simulink model "ECU_AEMACE"  (R2021b)
settings: Solver=FixedStepDiscrete  StartTime=0.0  StopTime=inf  RelTol=1e-3
undefined symbols (not defined in the file or in its folder): IO682
libraries: speedgoatlib_IO682 x38, simulink x1
settings Model: Creator=ACH  LastModifiedBy=angel
settings SolverCC: ConcurrentTasks=on  PositivePriorityOrder=on
settings OptimizationCC: BlockReduction=off  OptimizeBlockIOStorage=off
settings DebuggingCC: TasksWithSamePriorityMsg=none
settings HardwareCC: ProdBitPerLong=64  ProdLongLongMode=on  ProdHWDeviceType=Intel->x86-64 (Linux 64)
settings RTWCC: Description=Simulink Real-Time  SystemTargetFile=slrealtime.tlc  TemplateMakefile=slrealtime_default_tmf  Toolchain=Simulink Real-Time Toolchain  BuildConfiguration=Faster Runs  CodeExecutionProfiling=on  TargetLang=C++
settings SimulinkRealTimeTargetCC: UseGCCFastMath=on

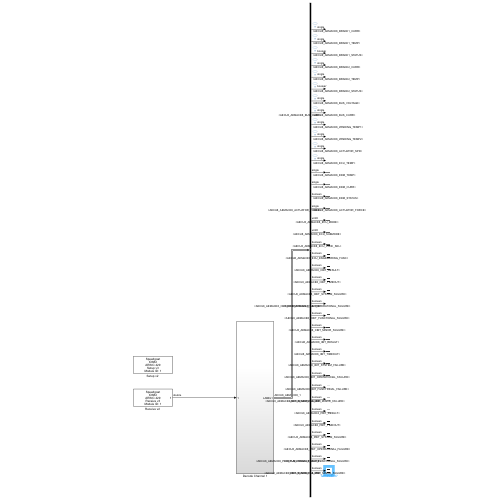
[thumbnail: Simulink's stored preview of the top-level diagram]
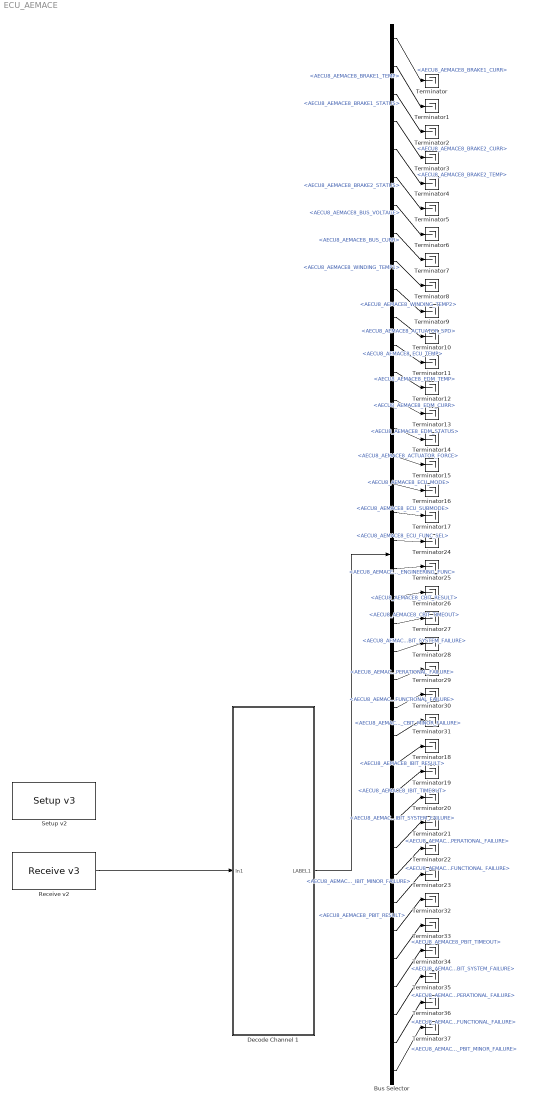
== system ECU_AEMACE ==
  Bus Selector : BusSelector  OutputSignals=AECU8_AEMACE8_BRAKE1_CURR,AECU8_AEMACE8_BRAKE1_TEMP,AECU8_AEMACE8_BRAKE1_STATUS,AECU8_AEMACE8_BRAKE2_CURR,AECU8_AEMACE8_BRAKE2_TEMP,AECU8_AEMACE8_BRAKE2_STATUS,AECU8_AEMACE8_BUS_VOLTAGE,AECU8_AEMACE8_BUS_CURR,AECU8_AEMACE8_WINDING_TEMP1,AECU8_AEMACE8_WINDING_TEMP2,AECU8_AEMACE8_ACTUATOR_SPD,AECU8_AEMACE8_ECU_TEMP,AECU8_AEMACE8_EDM_TEMP,AECU8_AEMACE8_EDM_CURR,AECU8_AEMACE8_EDM_STATUS,AECU8_AEMACE8_ACTUATOR_FORCE,AECU8_AEMACE8_ECU_MODE,AECU8_AEMACE8_ECU_SUBMODE,AECU8_AEMACE8_ECU_FUNC_SEL,AECU8_AEMACE8_ECU_ENGINEERING_FUNC,AECU8_AEMACE8_CBIT_RESULT,AECU8_AEMACE8_CBIT_TIMEOUT,AECU8_AEMACE8_CBIT_SYSTEM_FAILURE,AECU8_AEMACE8_CBIT_OPERATIONAL_FAILURE,AECU8_AEMACE8_CBIT_FUNCTIONAL_FAILURE,AECU8_AEMACE8_CBIT_MINOR_FAILURE,AECU8_AEMACE8_IBIT_RESULT,AECU8_AEMACE8_IBIT_TIMEOUT,AECU8_AEMACE8_IBIT_SYSTEM_FAILURE,AECU8_AEMACE8_IBIT_OPERATIONAL_FAILURE,AECU8_AEMACE8_IBIT_FUNCTIONAL_FAILURE,AECU8_AEMACE8_IBIT_MINOR_FAILURE,AECU8_AEMACE8_PBIT_RESULT,AECU8_AEMACE8_PBIT_TIMEOUT,AECU8_AEMACE8_PBIT_SYSTEM_FAILURE,AECU8_AEMACE8_PBIT_OPERATIONAL_FAILURE,AECU8_AEMACE8_PBIT_FUNCTIONAL_FAILURE,AECU8_AEMACE8_PBIT_MINOR_FAILURE
  Decode Channel 1 : Subsystem
  "Receive v2 " : speedgoatlib_IO682/Receive v3   parModuleId=1  parChannel=1  parMaxWords=10  parMinWords=1  parSampleTime=8e-3
      settings: SourceProductName=Speedgoat I/O Blockset
  "Setup v2 " : speedgoatlib_IO682/Setup v3   parModuleId=1  parBoardVariant=IO682-16-16  parPciSlot=-1  parTimerCount=4000*16  parChannelMode=Manual  parInBitRate1=100000  parInBufferMode1=Individual  parInEnable1=on  parInParity1=off  parInInternalWrap1=off  parInBitRate2=100000  parInBufferMode2=Individual  parInEnable2=on  parInParity2=on  parInInternalWrap2=off  parInBitRate3=100000  parInBufferMode3=Individual  parInEnable3=on  parInParity3=on  parInInternalWrap3=off  parInBitRate4=100000  parInBufferMode4=Individual  parInEnable4=on  parInParity4=on  parInInternalWrap4=off  parInBitRate5=100000  parInBufferMode5=Individual  parInEnable5=on  parInParity5=on  parInInternalWrap5=off  parInBitRate6=100000  parInBufferMode6=Individual  parInEnable6=on  parInParity6=on  parInInternalWrap6=off  parInBitRate7=100000  parInBufferMode7=Individual  parInEnable7=on  parInParity7=on  parInInternalWrap7=off  parInBitRate8=100000  parInBufferMode8=Individual  parInEnable8=on  parInParity8=on  parInInternalWrap8=off  parInBitRate9=100000  parInBufferMode9=Individual  parInEnable9=on  parInParity9=on  parInInternalWrap9=off  parInBitRate10=100000  parInBufferMode10=Individual  parInEnable10=on  parInParity10=on  parInInternalWrap10=off  parInBitRate11=100000  parInBufferMode11=Individual  parInEnable11=on  parInParity11=on  parInInternalWrap11=off  parInBitRate12=100000  parInBufferMode12=Individual  parInEnable12=on  parInParity12=on  parInInternalWrap12=off  parInBitRate13=100000  parInBufferMode13=Individual  parInEnable13=on  parInParity13=on  parInInternalWrap13=off  parInBitRate14=100000  parInBufferMode14=Individual  parInEnable14=on  parInParity14=on  parInInternalWrap14=off  parInBitRate15=100000  parInBufferMode15=Individual  parInEnable15=on  parInParity15=on  parInInternalWrap15=off  parInBitRate16=100000  parInBufferMode16=Individual  parInEnable16=on  parInParity16=on  parInInternalWrap16=off  parOutBitRate1=100000  parOutParity1=Odd  parOutProtocolError1=None  parOutEnable1=on  parOutBitRate2=100000  parOutParity2=Odd  parOutProtocolError2=None  parOutEnable2=on  parOutBitRate3=100000  parOutParity3=Odd  parOutProtocolError3=None  parOutEnable3=on  parOutBitRate4=100000  parOutParity4=Odd  parOutProtocolError4=None  parOutEnable4=on  parOutBitRate5=100000  parOutParity5=Odd  parOutProtocolError5=None  parOutEnable5=on  parOutBitRate6=100000  parOutParity6=Odd  parOutProtocolError6=None  parOutEnable6=on  parOutBitRate7=100000  parOutParity7=Odd  parOutProtocolError7=None  parOutEnable7=on  parOutBitRate8=100000  parOutParity8=Odd  parOutProtocolError8=None  parOutEnable8=on  parOutBitRate9=100000  parOutParity9=Odd  parOutProtocolError9=None  parOutEnable9=on  parOutBitRate10=100000  parOutParity10=Odd  parOutProtocolError10=None  parOutEnable10=on  parOutBitRate11=100000  parOutParity11=Odd  parOutProtocolError11=None  parOutEnable11=on  parOutBitRate12=100000  parOutParity12=Odd  parOutProtocolError12=None  parOutEnable12=on  parOutBitRate13=100000  parOutParity13=Odd  parOutProtocolError13=None  parOutEnable13=on  parOutBitRate14=100000  parOutParity14=Odd  parOutProtocolError14=None  parOutEnable14=on  parOutBitRate15=100000  parOutParity15=Odd  parOutProtocolError15=None  parOutEnable15=on  parOutBitRate16=100000  parOutParity16=Odd  parOutProtocolError16=None  parOutEnable16=on  parChConfigFile=''  parScheduleMode=Manual  parScheduledMsgConfigFile=''  parHwDeviceId=hex2dec('0830')  parTimeSource=Internal timer  parChInConfig=[158 8 7 8 1;158 8 7 7 1;158 8 7 7 1;158 8 7 7 1;158 8 7 7 1;158 8 7 7 1;158 8 7 7 1;158 8 7 7 1;158 8 7 7 1;158 8 7 7 1;158 8 7 7 1;158 8 7 7 1;158 8 7 7 1;158 8 7 7 1;158 8 7 7 1;158 8 7 7 1]  parChOutConfig=[158 0 4 7;158 0 4 7;158 0 4 7;158 0 4 7;158 0 4 7;158 0 4 7;158 0 4 7;158 0 4 7;158 0 4 7;158 0 4 7;158 0 4 7;158 0 4 7;158 0 4 7;158 0 4 7;158 0 4 7;158 0 4 7]  parScheduledMessages=0
      settings: SourceProductName=Speedgoat I/O Blockset
  Terminator{,1..37} (38 alike) : Terminator
  wires:
  "Receive v2 "/1 -> Decode Channel 1/1(In1)
  Decode Channel 1/1(LABEL1) -> Bus Selector/1
  Bus Selector/1 -> Terminator/1  "<AECU8_AEMACE8_BRAKE1_CURR>"
  Bus Selector/2 -> Terminator1/1  "<AECU8_AEMACE8_BRAKE1_TEMP>"
  Bus Selector/4 -> Terminator3/1  "<AECU8_AEMACE8_BRAKE2_CURR>"
  Bus Selector/3 -> Terminator2/1  "<AECU8_AEMACE8_BRAKE1_STATUS>"
  Bus Selector/7 -> Terminator6/1  "<AECU8_AEMACE8_BUS_VOLTAGE>"
  Bus Selector/8 -> Terminator7/1  "<AECU8_AEMACE8_BUS_CURR>"
  Bus Selector/6 -> Terminator5/1  "<AECU8_AEMACE8_BRAKE2_STATUS>"
  Bus Selector/5 -> Terminator4/1  "<AECU8_AEMACE8_BRAKE2_TEMP>"
  Bus Selector/13 -> Terminator12/1  "<AECU8_AEMACE8_EDM_TEMP>"
  Bus Selector/14 -> Terminator13/1  "<AECU8_AEMACE8_EDM_CURR>"
  Bus Selector/16 -> Terminator15/1  "<AECU8_AEMACE8_ACTUATOR_FORCE>"
  Bus Selector/15 -> Terminator14/1  "<AECU8_AEMACE8_EDM_STATUS>"
  Bus Selector/11 -> Terminator10/1  "<AECU8_AEMACE8_ACTUATOR_SPD>"
  Bus Selector/12 -> Terminator11/1  "<AECU8_AEMACE8_ECU_TEMP>"
  Bus Selector/10 -> Terminator9/1  "<AECU8_AEMACE8_WINDING_TEMP2>"
  Bus Selector/9 -> Terminator8/1  "<AECU8_AEMACE8_WINDING_TEMP1>"
  Bus Selector/25 -> Terminator30/1  "<AECU8_AEMACE8_CBIT_FUNCTIONAL_FAILURE>"
  Bus Selector/26 -> Terminator31/1  "<AECU8_AEMACE8_CBIT_MINOR_FAILURE>"
  Bus Selector/28 -> Terminator19/1  "<AECU8_AEMACE8_IBIT_TIMEOUT>"
  Bus Selector/27 -> Terminator18/1  "<AECU8_AEMACE8_IBIT_RESULT>"
  Bus Selector/31 -> Terminator22/1  "<AECU8_AEMACE8_IBIT_FUNCTIONAL_FAILURE>"
  Bus Selector/32 -> Terminator23/1  "<AECU8_AEMACE8_IBIT_MINOR_FAILURE>"
  Bus Selector/30 -> Terminator21/1  "<AECU8_AEMACE8_IBIT_OPERATIONAL_FAILURE>"
  Bus Selector/29 -> Terminator20/1  "<AECU8_AEMACE8_IBIT_SYSTEM_FAILURE>"
  Bus Selector/21 -> Terminator26/1  "<AECU8_AEMACE8_CBIT_RESULT>"
  Bus Selector/22 -> Terminator27/1  "<AECU8_AEMACE8_CBIT_TIMEOUT>"
  Bus Selector/24 -> Terminator29/1  "<AECU8_AEMACE8_CBIT_OPERATIONAL_FAILURE>"
  Bus Selector/23 -> Terminator28/1  "<AECU8_AEMACE8_CBIT_SYSTEM_FAILURE>"
  Bus Selector/19 -> Terminator24/1  "<AECU8_AEMACE8_ECU_FUNC_SEL>"
  Bus Selector/20 -> Terminator25/1  "<AECU8_AEMACE8_ECU_ENGINEERING_FUNC>"
  Bus Selector/18 -> Terminator17/1  "<AECU8_AEMACE8_ECU_SUBMODE>"
  Bus Selector/17 -> Terminator16/1  "<AECU8_AEMACE8_ECU_MODE>"
  Bus Selector/34 -> Terminator33/1  "<AECU8_AEMACE8_PBIT_TIMEOUT>"
  Bus Selector/35 -> Terminator34/1  "<AECU8_AEMACE8_PBIT_SYSTEM_FAILURE>"
  Bus Selector/37 -> Terminator36/1  "<AECU8_AEMACE8_PBIT_FUNCTIONAL_FAILURE>"
  Bus Selector/36 -> Terminator35/1  "<AECU8_AEMACE8_PBIT_OPERATIONAL_FAILURE>"
  Bus Selector/33 -> Terminator32/1  "<AECU8_AEMACE8_PBIT_RESULT>"
  Bus Selector/38 -> Terminator37/1  "<AECU8_AEMACE8_PBIT_MINOR_FAILURE>"

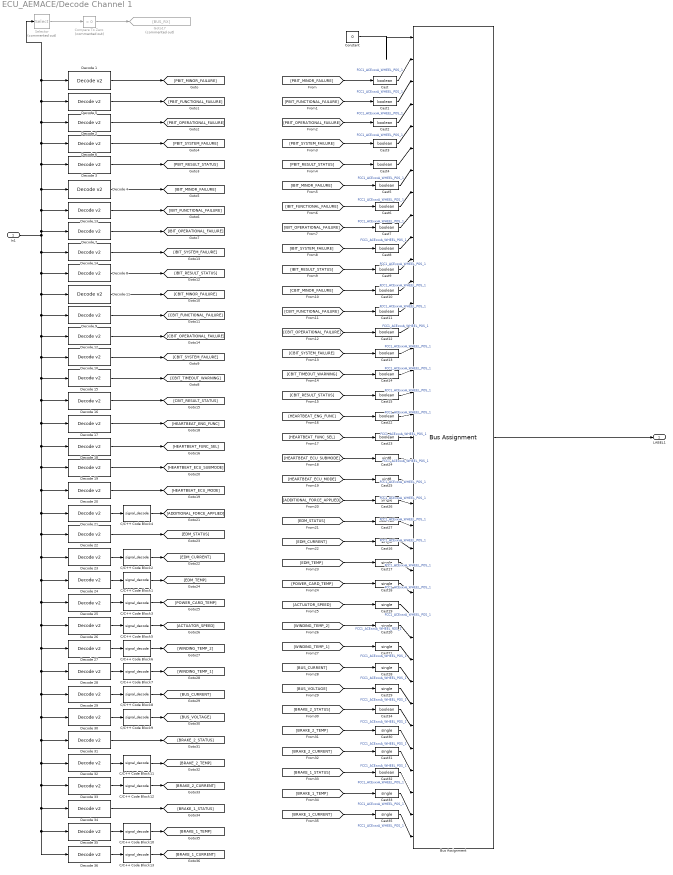
== system ECU_AEMACE/Decode Channel 1 ==
  In1 : Inport
  Bus Assignment : BusAssignment  AssignedSignals=AECU8_AEMACE8_PBIT_MINOR_FAILURE,AECU8_AEMACE8_PBIT_FUNCTIONAL_FAILURE,AECU8_AEMACE8_PBIT_OPERATIONAL_FAILURE,AECU8_AEMACE8_PBIT_SYSTEM_FAILURE,AECU8_AEMACE8_PBIT_RESULT,AECU8_AEMACE8_IBIT_MINOR_FAILURE,AECU8_AEMACE8_IBIT_FUNCTIONAL_FAILURE,AECU8_AEMACE8_IBIT_OPERATIONAL_FAILURE,AECU8_AEMACE8_IBIT_SYSTEM_FAILURE,AECU8_AEMACE8_IBIT_RESULT,AECU8_AEMACE8_CBIT_MINOR_FAILURE,AECU8_AEMACE8_CBIT_FUNCTIONAL_FAILURE,AECU8_AEMACE8_CBIT_OPERATIONAL_FAILURE,AECU8_AEMACE8_CBIT_SYSTEM_FAILURE,AECU8_AEMACE8_CBIT_TIMEOUT,AECU8_AEMACE8_CBIT_RESULT,AECU8_AEMACE8_ECU_ENGINEERING_FUNC,AECU8_AEMACE8_ECU_FUNC_SEL,AECU8_AEMACE8_ECU_SUBMODE,AECU8_AEMACE8_ECU_MODE,AECU8_AEMACE8_ACTUATOR_FORCE,AECU8_AEMACE8_EDM_STATUS,AECU8_AEMACE8_EDM_CURR,AECU8_AEMACE8_EDM_TEMP,AECU8_AEMACE8_ECU_TEMP,AECU8_AEMACE8_ACTUATOR_SPD,AECU8_AEMACE8_WINDING_TEMP2,AECU8_AEMACE8_WINDING_TEMP1,AECU8_AEMACE8_BUS_CURR,AECU8_AEMACE8_BUS_VOLTAGE,AECU8_AEMACE8_BRAKE2_STATUS,AECU8_AEMACE8_BRAKE2_TEMP,AECU8_AEMACE8_BRAKE2_CURR,AECU8_AEMACE8_BRAKE1_STATUS,AECU8_AEMACE8_BRAKE1_TEMP,AECU8_AEMACE8_BRAKE1_CURR
  C/C++ Code Block1 : S-Function  FunctionName=signal_decode  Parameters=1,0,boolean(1),boolean(0),uint32(9)  SFunctionModules=signal_decode_wrapper  SFunctionDeploymentMode=off  EnableBusSupport=off  mask(S-Function Builder){}
      mask help: Simulink:masks:SFunctionBuilder_MD
      mask init:
      | val = [[.9  0.75 0.75 1 1 .9 .9 1]',[1 1 0.75 0.75 .9 .9 1 .9]'];try , sys = get_param(gcb,'SfunBuilderFcnName');if isempty(sys), sys = get_param(gcb,'FunctionName'); end,catch, sys = get_param(gcb,'FunctionName'); end
      settings: CopyFcn=set_param(gcbh,'LinkStatus','none')  OpenFcn=sfunctionwizard(gcbh)
      mask Display: plot(val(:,1),val(:,2)),disp(sys),port_label('input',1,'data'),port_label('output',1,'out')
  C/C++ Code Block10 : S-Function  FunctionName=signal_decode  Parameters=1,0,boolean(1),boolean(0),uint32(9)  SFunctionModules=signal_decode_wrapper  SFunctionDeploymentMode=off  EnableBusSupport=off  mask(S-Function Builder){}
      mask help: Simulink:masks:SFunctionBuilder_MD
      mask init: same as ECU_AEMACE/Decode Channel 1/C/C++ Code Block1
      settings: CopyFcn=set_param(gcbh,'LinkStatus','none')  OpenFcn=sfunctionwizard(gcbh)
      mask Display: plot(val(:,1),val(:,2)),disp(sys),port_label('input',1,'data'),port_label('output',1,'out')
  C/C++ Code Block11 : S-Function  FunctionName=signal_decode  Parameters=1,0,boolean(1),boolean(0),uint32(9)  SFunctionModules=signal_decode_wrapper  SFunctionDeploymentMode=off  EnableBusSupport=off  mask(S-Function Builder){}
      mask help: Simulink:masks:SFunctionBuilder_MD
      mask init: same as ECU_AEMACE/Decode Channel 1/C/C++ Code Block1
      settings: CopyFcn=set_param(gcbh,'LinkStatus','none')  OpenFcn=sfunctionwizard(gcbh)
      mask Display: plot(val(:,1),val(:,2)),disp(sys),port_label('input',1,'data'),port_label('output',1,'out')
  C/C++ Code Block12 : S-Function  FunctionName=signal_decode  Parameters=0.01,0,boolean(1),boolean(0),uint32(9)  SFunctionModules=signal_decode_wrapper  SFunctionDeploymentMode=off  EnableBusSupport=off  mask(S-Function Builder){}
      mask help: Simulink:masks:SFunctionBuilder_MD
      mask init: same as ECU_AEMACE/Decode Channel 1/C/C++ Code Block1
      settings: CopyFcn=set_param(gcbh,'LinkStatus','none')  OpenFcn=sfunctionwizard(gcbh)
      mask Display: plot(val(:,1),val(:,2)),disp(sys),port_label('input',1,'data'),port_label('output',1,'out')
  C/C++ Code Block13 : S-Function  FunctionName=signal_decode  Parameters=0.01,0,boolean(1),boolean(0),uint32(9)  SFunctionModules=signal_decode_wrapper  SFunctionDeploymentMode=off  EnableBusSupport=off  mask(S-Function Builder){}
      mask help: Simulink:masks:SFunctionBuilder_MD
      mask init: same as ECU_AEMACE/Decode Channel 1/C/C++ Code Block1
      settings: CopyFcn=set_param(gcbh,'LinkStatus','none')  OpenFcn=sfunctionwizard(gcbh)
      mask Display: plot(val(:,1),val(:,2)),disp(sys),port_label('input',1,'data'),port_label('output',1,'out')
  C/C++ Code Block2 : S-Function  FunctionName=signal_decode  Parameters=0.1,0,boolean(1),boolean(0),uint32(9)  SFunctionModules=signal_decode_wrapper  SFunctionDeploymentMode=off  EnableBusSupport=off  mask(S-Function Builder){}
      mask help: Simulink:masks:SFunctionBuilder_MD
      mask init: same as ECU_AEMACE/Decode Channel 1/C/C++ Code Block1
      settings: CopyFcn=set_param(gcbh,'LinkStatus','none')  OpenFcn=sfunctionwizard(gcbh)
      mask Display: plot(val(:,1),val(:,2)),disp(sys),port_label('input',1,'data'),port_label('output',1,'out')
  C/C++ Code Block3 : S-Function  FunctionName=signal_decode  Parameters=1,0,boolean(1),boolean(0),uint32(9)  SFunctionModules=signal_decode_wrapper  SFunctionDeploymentMode=off  EnableBusSupport=off  mask(S-Function Builder){}
      mask help: Simulink:masks:SFunctionBuilder_MD
      mask init: same as ECU_AEMACE/Decode Channel 1/C/C++ Code Block1
      settings: CopyFcn=set_param(gcbh,'LinkStatus','none')  OpenFcn=sfunctionwizard(gcbh)
      mask Display: plot(val(:,1),val(:,2)),disp(sys),port_label('input',1,'data'),port_label('output',1,'out')
  C/C++ Code Block4 : S-Function  FunctionName=signal_decode  Parameters=1,0,boolean(1),boolean(0),uint32(8)  SFunctionModules=signal_decode_wrapper  SFunctionDeploymentMode=off  EnableBusSupport=off  mask(S-Function Builder){}
      mask help: Simulink:masks:SFunctionBuilder_MD
      mask init: same as ECU_AEMACE/Decode Channel 1/C/C++ Code Block1
      settings: CopyFcn=set_param(gcbh,'LinkStatus','none')  OpenFcn=sfunctionwizard(gcbh)
      mask Display: plot(val(:,1),val(:,2)),disp(sys),port_label('input',1,'data'),port_label('output',1,'out')
  C/C++ Code Block5 : S-Function  FunctionName=signal_decode  Parameters=5/128,0,boolean(1),boolean(0),uint32(16)  SFunctionModules=signal_decode_wrapper  SFunctionDeploymentMode=off  EnableBusSupport=off  mask(S-Function Builder){}
      mask help: Simulink:masks:SFunctionBuilder_MD
      mask init: same as ECU_AEMACE/Decode Channel 1/C/C++ Code Block1
      settings: CopyFcn=set_param(gcbh,'LinkStatus','none')  OpenFcn=sfunctionwizard(gcbh)
      mask Display: plot(val(:,1),val(:,2)),disp(sys),port_label('input',1,'data'),port_label('output',1,'out')
  C/C++ Code Block6 : S-Function  FunctionName=signal_decode  Parameters=1,0,boolean(1),boolean(0),uint32(9)  SFunctionModules=signal_decode_wrapper  SFunctionDeploymentMode=off  EnableBusSupport=off  mask(S-Function Builder){}
      mask help: Simulink:masks:SFunctionBuilder_MD
      mask init: same as ECU_AEMACE/Decode Channel 1/C/C++ Code Block1
      settings: CopyFcn=set_param(gcbh,'LinkStatus','none')  OpenFcn=sfunctionwizard(gcbh)
      mask Display: plot(val(:,1),val(:,2)),disp(sys),port_label('input',1,'data'),port_label('output',1,'out')
  C/C++ Code Block7 : S-Function  FunctionName=signal_decode  Parameters=1,0,boolean(1),boolean(0),uint32(9)  SFunctionModules=signal_decode_wrapper  SFunctionDeploymentMode=off  EnableBusSupport=off  mask(S-Function Builder){}
      mask help: Simulink:masks:SFunctionBuilder_MD
      mask init: same as ECU_AEMACE/Decode Channel 1/C/C++ Code Block1
      settings: CopyFcn=set_param(gcbh,'LinkStatus','none')  OpenFcn=sfunctionwizard(gcbh)
      mask Display: plot(val(:,1),val(:,2)),disp(sys),port_label('input',1,'data'),port_label('output',1,'out')
  C/C++ Code Block8 : S-Function  FunctionName=signal_decode  Parameters=1,0,boolean(1),boolean(0),uint32(7)  SFunctionModules=signal_decode_wrapper  SFunctionDeploymentMode=off  EnableBusSupport=off  mask(S-Function Builder){}
      mask help: Simulink:masks:SFunctionBuilder_MD
      mask init: same as ECU_AEMACE/Decode Channel 1/C/C++ Code Block1
      settings: CopyFcn=set_param(gcbh,'LinkStatus','none')  OpenFcn=sfunctionwizard(gcbh)
      mask Display: plot(val(:,1),val(:,2)),disp(sys),port_label('input',1,'data'),port_label('output',1,'out')
  C/C++ Code Block9 : S-Function  FunctionName=signal_decode  Parameters=1,0,boolean(1),boolean(0),uint32(10)  SFunctionModules=signal_decode_wrapper  SFunctionDeploymentMode=off  EnableBusSupport=off  mask(S-Function Builder){}
      mask help: Simulink:masks:SFunctionBuilder_MD
      mask init: same as ECU_AEMACE/Decode Channel 1/C/C++ Code Block1
      settings: CopyFcn=set_param(gcbh,'LinkStatus','none')  OpenFcn=sfunctionwizard(gcbh)
      mask Display: plot(val(:,1),val(:,2)),disp(sys),port_label('input',1,'data'),port_label('output',1,'out')
  Cast{,1..15,22..23,27,32,34} (21 alike) : DataTypeConversion  OutDataTypeStr=boolean
  Cast{16..21,26,28..31,33,35} (13 alike) : DataTypeConversion  OutDataTypeStr=single
  Cast24 : DataTypeConversion  OutDataTypeStr=uint8
  Cast25 : DataTypeConversion  OutDataTypeStr=uint8
  Compare To Zero : simulink/Logic and Bit Operations/Compare To Zero  Commented=on  relop=>  OutDataTypeStr=boolean
  Constant : Constant  Value=0  OutDataTypeStr=Bus: AECU8_AEMACE8_1  SampleTime=0.008
  Decode 1 : speedgoatlib_IO682/Decode v2   parMode=Custom Data Type  parLabel=223  parDataType=[2]  parResolution=[4096]  parSyncMask=hex2dec('0x0')  parSyncValue=hex2dec('0x0')  parCustomDataType=Discrete  parDataLSB=11  parDataMSB=18  parBitPosition=[25]  parScaleBNR=1  parExponent=8  parMantissa=14  parTimeTags=off  parHoldLastVal=on  parStatus=off
      settings: SourceProductName=Simulink Real-Time: Speedgoat I/O Blockset
  Decode 10 : speedgoatlib_IO682/Decode v2   parMode=Custom Data Type  parLabel=221  parDataType=[3]  parResolution=[.1]  parSyncMask=hex2dec('0x0')  parSyncValue=hex2dec('0x0')  parCustomDataType=Discrete  parDataLSB=24  parDataMSB=27  parBitPosition=[27]  parScaleBNR=1  parExponent=8  parMantissa=14  parTimeTags=off  parHoldLastVal=on  parStatus=off
      settings: SourceProductName=Simulink Real-Time: Speedgoat I/O Blockset
  Decode 11 : speedgoatlib_IO682/Decode v2   parMode=Custom Data Type  parLabel=221  parDataType=[2]  parResolution=[4096]  parSyncMask=hex2dec('0x0')  parSyncValue=hex2dec('0x0')  parCustomDataType=Discrete  parDataLSB=11  parDataMSB=18  parBitPosition=[24]  parScaleBNR=1  parExponent=8  parMantissa=14  parTimeTags=off  parHoldLastVal=on  parStatus=off
      settings: SourceProductName=Simulink Real-Time: Speedgoat I/O Blockset
  Decode 12 : speedgoatlib_IO682/Decode v2   parMode=Custom Data Type  parLabel=221  parDataType=[3]  parResolution=[.1]  parSyncMask=hex2dec('0x0')  parSyncValue=hex2dec('0x0')  parCustomDataType=Discrete  parDataLSB=11  parDataMSB=20  parBitPosition=[26]  parScaleBNR=1  parExponent=8  parMantissa=14  parTimeTags=off  parHoldLastVal=on  parStatus=off
      settings: SourceProductName=Simulink Real-Time: Speedgoat I/O Blockset
  Decode 13 : speedgoatlib_IO682/Decode v2   parMode=Custom Data Type  parLabel=222  parDataType=[3]  parResolution=[.1]  parSyncMask=hex2dec('0x0')  parSyncValue=hex2dec('0x0')  parCustomDataType=Discrete  parDataLSB=19  parDataMSB=26  parBitPosition=[26]  parScaleBNR=1  parExponent=8  parMantissa=14  parTimeTags=off  parHoldLastVal=on  parStatus=off
      settings: SourceProductName=Simulink Real-Time: Speedgoat I/O Blockset
  Decode 14 : speedgoatlib_IO682/Decode v2   parMode=Custom Data Type  parLabel=222  parDataType=[3]  parResolution=[.1]  parSyncMask=hex2dec('0x0')  parSyncValue=hex2dec('0x0')  parCustomDataType=Discrete  parDataLSB=24  parDataMSB=27  parBitPosition=[28]  parScaleBNR=1  parExponent=8  parMantissa=14  parTimeTags=off  parHoldLastVal=on  parStatus=off
      settings: SourceProductName=Simulink Real-Time: Speedgoat I/O Blockset
  Decode 15 : speedgoatlib_IO682/Decode v2   parMode=Custom Data Type  parLabel=221  parDataType=[3]  parResolution=[.1]  parSyncMask=hex2dec('0x0')  parSyncValue=hex2dec('0x0')  parCustomDataType=Discrete  parDataLSB=24  parDataMSB=27  parBitPosition=[28]  parScaleBNR=1  parExponent=8  parMantissa=14  parTimeTags=off  parHoldLastVal=on  parStatus=off
      settings: SourceProductName=Simulink Real-Time: Speedgoat I/O Blockset
  Decode 16 : speedgoatlib_IO682/Decode v2   parMode=Custom Data Type  parLabel=222  parDataType=[3]  parResolution=[.1]  parSyncMask=hex2dec('0x0')  parSyncValue=hex2dec('0x0')  parCustomDataType=Discrete  parDataLSB=24  parDataMSB=27  parBitPosition=[29]  parScaleBNR=1  parExponent=8  parMantissa=14  parTimeTags=off  parHoldLastVal=on  parStatus=off
      settings: SourceProductName=Simulink Real-Time: Speedgoat I/O Blockset
  Decode 17 : speedgoatlib_IO682/Decode v2   parMode=Custom Data Type  parLabel=220  parDataType=[3]  parResolution=[.1]  parSyncMask=hex2dec('0x0')  parSyncValue=hex2dec('0x0')  parCustomDataType=Discrete  parDataLSB=24  parDataMSB=27  parBitPosition=[11]  parScaleBNR=1  parExponent=8  parMantissa=14  parTimeTags=off  parHoldLastVal=on  parStatus=off
      settings: SourceProductName=Simulink Real-Time: Speedgoat I/O Blockset
  Decode 18 : speedgoatlib_IO682/Decode v2   parMode=Custom Data Type  parLabel=220  parDataType=[3]  parResolution=[.1]  parSyncMask=hex2dec('0x0')  parSyncValue=hex2dec('0x0')  parCustomDataType=Discrete  parDataLSB=24  parDataMSB=27  parBitPosition=[12]  parScaleBNR=1  parExponent=8  parMantissa=14  parTimeTags=off  parHoldLastVal=on  parStatus=off
      settings: SourceProductName=Simulink Real-Time: Speedgoat I/O Blockset
  Decode 19 : speedgoatlib_IO682/Decode v2   parMode=Custom Data Type  parLabel=220  parDataType=[3]  parResolution=[.1]  parSyncMask=hex2dec('0x0')  parSyncValue=hex2dec('0x0')  parCustomDataType=Raw  parDataLSB=24  parDataMSB=26  parBitPosition=[11]  parScaleBNR=1  parExponent=8  parMantissa=14  parTimeTags=off  parHoldLastVal=on  parStatus=off
      settings: SourceProductName=Simulink Real-Time: Speedgoat I/O Blockset
  Decode 2 : speedgoatlib_IO682/Decode v2   parMode=Custom Data Type  parLabel=223  parDataType=[3]  parResolution=[.1]  parSyncMask=hex2dec('0x0')  parSyncValue=hex2dec('0x0')  parCustomDataType=Discrete  parDataLSB=11  parDataMSB=20  parBitPosition=[27]  parScaleBNR=1  parExponent=8  parMantissa=14  parTimeTags=off  parHoldLastVal=on  parStatus=off
      settings: SourceProductName=Simulink Real-Time: Speedgoat I/O Blockset
  Decode 20 : speedgoatlib_IO682/Decode v2   parMode=Custom Data Type  parLabel=220  parDataType=[3]  parResolution=[.1]  parSyncMask=hex2dec('0x0')  parSyncValue=hex2dec('0x0')  parCustomDataType=Raw  parDataLSB=27  parDataMSB=29  parBitPosition=[12]  parScaleBNR=1  parExponent=8  parMantissa=14  parTimeTags=off  parHoldLastVal=on  parStatus=off
      settings: SourceProductName=Simulink Real-Time: Speedgoat I/O Blockset
  Decode 21 : speedgoatlib_IO682/Decode v2   parMode=Custom Data Type  parLabel=217  parDataType=[3]  parResolution=[.1]  parSyncMask=hex2dec('0x0')  parSyncValue=hex2dec('0x0')  parCustomDataType=Raw  parDataLSB=22  parDataMSB=29  parBitPosition=[12]  parScaleBNR=1  parExponent=8  parMantissa=14  parTimeTags=off  parHoldLastVal=on  parStatus=off
      settings: SourceProductName=Simulink Real-Time: Speedgoat I/O Blockset
  Decode 22 : speedgoatlib_IO682/Decode v2   parMode=Custom Data Type  parLabel=216  parDataType=[3]  parResolution=[.1]  parSyncMask=hex2dec('0x0')  parSyncValue=hex2dec('0x0')  parCustomDataType=Discrete  parDataLSB=24  parDataMSB=26  parBitPosition=[11]  parScaleBNR=1  parExponent=8  parMantissa=14  parTimeTags=off  parHoldLastVal=on  parStatus=off
      settings: SourceProductName=Simulink Real-Time: Speedgoat I/O Blockset
  Decode 23 : speedgoatlib_IO682/Decode v2   parMode=Custom Data Type  parLabel=216  parDataType=[3]  parResolution=[.1]  parSyncMask=hex2dec('0x0')  parSyncValue=hex2dec('0x0')  parCustomDataType=Raw  parDataLSB=12  parDataMSB=20  parBitPosition=[12]  parScaleBNR=1  parExponent=8  parMantissa=14  parTimeTags=off  parHoldLastVal=on  parStatus=off
      settings: SourceProductName=Simulink Real-Time: Speedgoat I/O Blockset
  Decode 24 : speedgoatlib_IO682/Decode v2   parMode=Custom Data Type  parLabel=216  parDataType=[3]  parResolution=[.1]  parSyncMask=hex2dec('0x0')  parSyncValue=hex2dec('0x0')  parCustomDataType=Raw  parDataLSB=21  parDataMSB=29  parBitPosition=[12]  parScaleBNR=1  parExponent=8  parMantissa=14  parTimeTags=off  parHoldLastVal=on  parStatus=off
      settings: SourceProductName=Simulink Real-Time: Speedgoat I/O Blockset
  Decode 25 : speedgoatlib_IO682/Decode v2   parMode=Custom Data Type  parLabel=215  parDataType=[3]  parResolution=[.1]  parSyncMask=hex2dec('0x0')  parSyncValue=hex2dec('0x0')  parCustomDataType=Raw  parDataLSB=21  parDataMSB=29  parBitPosition=[12]  parScaleBNR=1  parExponent=8  parMantissa=14  parTimeTags=off  parHoldLastVal=on  parStatus=off
      settings: SourceProductName=Simulink Real-Time: Speedgoat I/O Blockset
  Decode 26 : speedgoatlib_IO682/Decode v2   parMode=Custom Data Type  parLabel=214  parDataType=[3]  parResolution=[.1]  parSyncMask=hex2dec('0x0')  parSyncValue=hex2dec('0x0')  parCustomDataType=Raw  parDataLSB=14  parDataMSB=29  parBitPosition=[12]  parScaleBNR=1  parExponent=8  parMantissa=14  parTimeTags=off  parHoldLastVal=on  parStatus=off
      settings: SourceProductName=Simulink Real-Time: Speedgoat I/O Blockset
  Decode 27 : speedgoatlib_IO682/Decode v2   parMode=Custom Data Type  parLabel=213  parDataType=[3]  parResolution=[.1]  parSyncMask=hex2dec('0x0')  parSyncValue=hex2dec('0x0')  parCustomDataType=Raw  parDataLSB=12  parDataMSB=20  parBitPosition=[12]  parScaleBNR=1  parExponent=8  parMantissa=14  parTimeTags=off  parHoldLastVal=on  parStatus=off
      settings: SourceProductName=Simulink Real-Time: Speedgoat I/O Blockset
  Decode 28 : speedgoatlib_IO682/Decode v2   parMode=Custom Data Type  parLabel=213  parDataType=[3]  parResolution=[.1]  parSyncMask=hex2dec('0x0')  parSyncValue=hex2dec('0x0')  parCustomDataType=Raw  parDataLSB=21  parDataMSB=29  parBitPosition=[12]  parScaleBNR=1  parExponent=8  parMantissa=14  parTimeTags=off  parHoldLastVal=on  parStatus=off
      settings: SourceProductName=Simulink Real-Time: Speedgoat I/O Blockset
  Decode 29 : speedgoatlib_IO682/Decode v2   parMode=Custom Data Type  parLabel=212  parDataType=[3]  parResolution=[.1]  parSyncMask=hex2dec('0x0')  parSyncValue=hex2dec('0x0')  parCustomDataType=Raw  parDataLSB=13  parDataMSB=19  parBitPosition=[12]  parScaleBNR=1  parExponent=8  parMantissa=14  parTimeTags=off  parHoldLastVal=on  parStatus=off
      settings: SourceProductName=Simulink Real-Time: Speedgoat I/O Blockset
  Decode 3 : speedgoatlib_IO682/Decode v2   parMode=Custom Data Type  parLabel=223  parDataType=[3]  parResolution=[.1]  parSyncMask=hex2dec('0x0')  parSyncValue=hex2dec('0x0')  parCustomDataType=Discrete  parDataLSB=24  parDataMSB=27  parBitPosition=[29]  parScaleBNR=1  parExponent=8  parMantissa=14  parTimeTags=off  parHoldLastVal=on  parStatus=off
      settings: SourceProductName=Simulink Real-Time: Speedgoat I/O Blockset
  Decode 30 : speedgoatlib_IO682/Decode v2   parMode=Custom Data Type  parLabel=212  parDataType=[3]  parResolution=[.1]  parSyncMask=hex2dec('0x0')  parSyncValue=hex2dec('0x0')  parCustomDataType=Raw  parDataLSB=20  parDataMSB=29  parBitPosition=[12]  parScaleBNR=1  parExponent=8  parMantissa=14  parTimeTags=off  parHoldLastVal=on  parStatus=off
      settings: SourceProductName=Simulink Real-Time: Speedgoat I/O Blockset
  Decode 31 : speedgoatlib_IO682/Decode v2   parMode=Custom Data Type  parLabel=211  parDataType=[3]  parResolution=[.1]  parSyncMask=hex2dec('0x0')  parSyncValue=hex2dec('0x0')  parCustomDataType=Discrete  parDataLSB=21  parDataMSB=29  parBitPosition=[11]  parScaleBNR=1  parExponent=8  parMantissa=14  parTimeTags=off  parHoldLastVal=on  parStatus=off
      settings: SourceProductName=Simulink Real-Time: Speedgoat I/O Blockset
  Decode 32 : speedgoatlib_IO682/Decode v2   parMode=Custom Data Type  parLabel=211  parDataType=[3]  parResolution=[.1]  parSyncMask=hex2dec('0x0')  parSyncValue=hex2dec('0x0')  parCustomDataType=Raw  parDataLSB=12  parDataMSB=20  parBitPosition=[12]  parScaleBNR=1  parExponent=8  parMantissa=14  parTimeTags=off  parHoldLastVal=on  parStatus=off
      settings: SourceProductName=Simulink Real-Time: Speedgoat I/O Blockset
  Decode 33 : speedgoatlib_IO682/Decode v2   parMode=Custom Data Type  parLabel=211  parDataType=[3]  parResolution=[.1]  parSyncMask=hex2dec('0x0')  parSyncValue=hex2dec('0x0')  parCustomDataType=Raw  parDataLSB=21  parDataMSB=29  parBitPosition=[12]  parScaleBNR=1  parExponent=8  parMantissa=14  parTimeTags=off  parHoldLastVal=on  parStatus=off
      settings: SourceProductName=Simulink Real-Time: Speedgoat I/O Blockset
  Decode 34 : speedgoatlib_IO682/Decode v2   parMode=Custom Data Type  parLabel=210  parDataType=[3]  parResolution=[.1]  parSyncMask=hex2dec('0x0')  parSyncValue=hex2dec('0x0')  parCustomDataType=Discrete  parDataLSB=21  parDataMSB=29  parBitPosition=[11]  parScaleBNR=1  parExponent=8  parMantissa=14  parTimeTags=off  parHoldLastVal=on  parStatus=off
      settings: SourceProductName=Simulink Real-Time: Speedgoat I/O Blockset
  Decode 35 : speedgoatlib_IO682/Decode v2   parMode=Custom Data Type  parLabel=210  parDataType=[3]  parResolution=[.1]  parSyncMask=hex2dec('0x0')  parSyncValue=hex2dec('0x0')  parCustomDataType=Raw  parDataLSB=12  parDataMSB=20  parBitPosition=[12]  parScaleBNR=1  parExponent=8  parMantissa=14  parTimeTags=off  parHoldLastVal=on  parStatus=off
      settings: SourceProductName=Simulink Real-Time: Speedgoat I/O Blockset
  Decode 36 : speedgoatlib_IO682/Decode v2   parMode=Custom Data Type  parLabel=210  parDataType=[3]  parResolution=[.1]  parSyncMask=hex2dec('0x0')  parSyncValue=hex2dec('0x0')  parCustomDataType=Raw  parDataLSB=21  parDataMSB=29  parBitPosition=[12]  parScaleBNR=1  parExponent=8  parMantissa=14  parTimeTags=off  parHoldLastVal=on  parStatus=off
      settings: SourceProductName=Simulink Real-Time: Speedgoat I/O Blockset
  Decode 4 : speedgoatlib_IO682/Decode v2   parMode=Custom Data Type  parLabel=222  parDataType=[2]  parResolution=[4096]  parSyncMask=hex2dec('0x0')  parSyncValue=hex2dec('0x0')  parCustomDataType=Discrete  parDataLSB=11  parDataMSB=18  parBitPosition=[25]  parScaleBNR=1  parExponent=8  parMantissa=14  parTimeTags=off  parHoldLastVal=on  parStatus=off
      settings: SourceProductName=Simulink Real-Time: Speedgoat I/O Blockset
  Decode 5 : speedgoatlib_IO682/Decode v2   parMode=Custom Data Type  parLabel=223  parDataType=[3]  parResolution=[.1]  parSyncMask=hex2dec('0x0')  parSyncValue=hex2dec('0x0')  parCustomDataType=Discrete  parDataLSB=19  parDataMSB=26  parBitPosition=[26]  parScaleBNR=1  parExponent=8  parMantissa=14  parTimeTags=off  parHoldLastVal=on  parStatus=off
      settings: SourceProductName=Simulink Real-Time: Speedgoat I/O Blockset
  Decode 6 : speedgoatlib_IO682/Decode v2   parMode=Custom Data Type  parLabel=223  parDataType=[3]  parResolution=[.1]  parSyncMask=hex2dec('0x0')  parSyncValue=hex2dec('0x0')  parCustomDataType=Discrete  parDataLSB=24  parDataMSB=27  parBitPosition=[28]  parScaleBNR=1  parExponent=8  parMantissa=14  parTimeTags=off  parHoldLastVal=on  parStatus=off
      settings: SourceProductName=Simulink Real-Time: Speedgoat I/O Blockset
  Decode 7 : speedgoatlib_IO682/Decode v2   parMode=Custom Data Type  parLabel=222  parDataType=[3]  parResolution=[.1]  parSyncMask=hex2dec('0x0')  parSyncValue=hex2dec('0x0')  parCustomDataType=Discrete  parDataLSB=11  parDataMSB=20  parBitPosition=[27]  parScaleBNR=1  parExponent=8  parMantissa=14  parTimeTags=off  parHoldLastVal=on  parStatus=off
      settings: SourceProductName=Simulink Real-Time: Speedgoat I/O Blockset
  Decode 8 : speedgoatlib_IO682/Decode v2   parMode=Custom Data Type  parLabel=222  parDataType=[3]  parResolution=[.1]  parSyncMask=hex2dec('0x0')  parSyncValue=hex2dec('0x0')  parCustomDataType=Discrete  parDataLSB=24  parDataMSB=27  parBitPosition=[29]  parScaleBNR=1  parExponent=8  parMantissa=14  parTimeTags=off  parHoldLastVal=on  parStatus=off
      settings: SourceProductName=Simulink Real-Time: Speedgoat I/O Blockset
  Decode 9 : speedgoatlib_IO682/Decode v2   parMode=Custom Data Type  parLabel=221  parDataType=[3]  parResolution=[.1]  parSyncMask=hex2dec('0x0')  parSyncValue=hex2dec('0x0')  parCustomDataType=Discrete  parDataLSB=19  parDataMSB=26  parBitPosition=[25]  parScaleBNR=1  parExponent=8  parMantissa=14  parTimeTags=off  parHoldLastVal=on  parStatus=off
      settings: SourceProductName=Simulink Real-Time: Speedgoat I/O Blockset
  Goto17 : Goto  Commented=on  GotoTag=BUS_RX
  Selector : Selector  Commented=on  InputPortWidth=11  IndexOptions=Index vector (dialog)  Indices=[1]  OutputSizes=1
  LABEL1 : Outport
  wires:
  Decode 6/1 -> [PBIT_SYSTEM_FAILURE]
  [PBIT_MINOR_FAILURE] -> Cast/1
  Decode 1/1 -> [PBIT_MINOR_FAILURE]
  Selector/1 -> Compare To Zero/1
  Compare To Zero/1 -> Goto17/1
  Decode 5/1 -> [PBIT_FUNCTIONAL_FAILURE]
  Decode 2/1 -> [PBIT_OPERATIONAL_FAILURE]
  Bus Assignment/1 -> LABEL1/1
  Constant/1 -> Bus Assignment/1
  Decode 3/1 -> [PBIT_RESULT_STATUS]
  Decode 8/1 -> [IBIT_RESULT_STATUS]
  Decode 7/1 -> [IBIT_OPERATIONAL_FAILURE]
  Decode 13/1 -> [IBIT_FUNCTIONAL_FAILURE]
  Decode 4/1 -> [IBIT_MINOR_FAILURE]
  Decode 14/1 -> [IBIT_SYSTEM_FAILURE]
  Decode 10/1 -> [CBIT_SYSTEM_FAILURE]
  Decode 11/1 -> [CBIT_MINOR_FAILURE]
  Decode 9/1 -> [CBIT_FUNCTIONAL_FAILURE]
  Decode 12/1 -> [CBIT_OPERATIONAL_FAILURE]
  Decode 15/1 -> [CBIT_TIMEOUT_WARNING]
  Decode 16/1 -> [CBIT_RESULT_STATUS]
  Decode 18/1 -> [HEARTBEAT_FUNC_SEL]
  Decode 17/1 -> [HEARTBEAT_ENG_FUNC]
  Decode 19/1 -> [HEARTBEAT_ECU_SUBMODE]
  Decode 20/1 -> [HEARTBEAT_ECU_MODE]
  Decode 21/1 -> C/C++ Code Block4/1
  C/C++ Code Block4/1 -> [ADDITIONAL_FORCE_APPLIED]
  C/C++ Code Block1/1 -> [EDM_TEMP]
  Decode 24/1 -> C/C++ Code Block1/1
  Decode 23/1 -> C/C++ Code Block2/1
  Decode 22/1 -> [EDM_STATUS]
  C/C++ Code Block2/1 -> [EDM_CURRENT]
  Decode 25/1 -> C/C++ Code Block3/1
  C/C++ Code Block3/1 -> [POWER_CARD_TEMP]
  C/C++ Code Block5/1 -> [ACTUATOR_SPEED]
  Decode 26/1 -> C/C++ Code Block5/1
  Decode 28/1 -> C/C++ Code Block7/1
  C/C++ Code Block7/1 -> [WINDING_TEMP_1]
  C/C++ Code Block6/1 -> [WINDING_TEMP_2]
  Decode 27/1 -> C/C++ Code Block6/1
  Decode 29/1 -> C/C++ Code Block8/1
  C/C++ Code Block8/1 -> [BUS_CURRENT]
  C/C++ Code Block9/1 -> [BUS_VOLTAGE]
  Decode 30/1 -> C/C++ Code Block9/1
  Decode 33/1 -> C/C++ Code Block12/1
  C/C++ Code Block12/1 -> [BRAKE_2_CURRENT]
  C/C++ Code Block11/1 -> [BRAKE_2_TEMP]
  Decode 32/1 -> C/C++ Code Block11/1
  Decode 31/1 -> [BRAKE_2_STATUS]
  Decode 34/1 -> [BRAKE_1_STATUS]
  Decode 35/1 -> C/C++ Code Block10/1
  C/C++ Code Block10/1 -> [BRAKE_1_TEMP]
  C/C++ Code Block13/1 -> [BRAKE_1_CURRENT]
  Decode 36/1 -> C/C++ Code Block13/1
  In1/1 -> Decode 7/1, Decode 13/1, Decode 4/1, Decode 3/1, Decode 6/1, Decode 2/1, Decode 5/1, Selector/1, Decode 1/1, Decode 14/1, Decode 8/1, Decode 9/1, Decode 12/1, Decode 10/1, Decode 15/1, Decode 19/1, Decode 23/1, Decode 27/1, Decode 31/1, Decode 32/1, Decode 36/1, Decode 35/1, Decode 34/1, Decode 33/1, Decode 30/1, Decode 29/1, Decode 28/1, Decode 26/1, Decode 25/1, Decode 24/1, Decode 22/1, Decode 21/1, Decode 20/1, Decode 18/1, Decode 17/1, Decode 16/1, Decode 11/1
  [PBIT_FUNCTIONAL_FAILURE] -> Cast1/1
  [PBIT_OPERATIONAL_FAILURE] -> Cast2/1
  [PBIT_SYSTEM_FAILURE] -> Cast3/1
  [PBIT_RESULT_STATUS] -> Cast4/1
  [IBIT_MINOR_FAILURE] -> Cast5/1
  [IBIT_FUNCTIONAL_FAILURE] -> Cast6/1
  [IBIT_OPERATIONAL_FAILURE] -> Cast7/1
  [IBIT_SYSTEM_FAILURE] -> Cast8/1
  [IBIT_RESULT_STATUS] -> Cast9/1
  [CBIT_TIMEOUT_WARNING] -> Cast14/1
  [CBIT_SYSTEM_FAILURE] -> Cast13/1
  [CBIT_OPERATIONAL_FAILURE] -> Cast12/1
  [CBIT_FUNCTIONAL_FAILURE] -> Cast11/1
  [CBIT_MINOR_FAILURE] -> Cast10/1
  [CBIT_RESULT_STATUS] -> Cast15/1
  [HEARTBEAT_ENG_FUNC] -> Cast22/1
  [HEARTBEAT_FUNC_SEL] -> Cast23/1
  [HEARTBEAT_ECU_SUBMODE] -> Cast24/1
  [HEARTBEAT_ECU_MODE] -> Cast25/1
  [ADDITIONAL_FORCE_APPLIED] -> Cast26/1
  [EDM_STATUS] -> Cast27/1
  [EDM_CURRENT] -> Cast16/1
  [EDM_TEMP] -> Cast17/1
  [POWER_CARD_TEMP] -> Cast18/1
  [ACTUATOR_SPEED] -> Cast19/1
  [WINDING_TEMP_2] -> Cast20/1
  [WINDING_TEMP_1] -> Cast21/1
  [BUS_CURRENT] -> Cast28/1
  [BUS_VOLTAGE] -> Cast29/1
  [BRAKE_2_STATUS] -> Cast34/1
  [BRAKE_1_CURRENT] -> Cast35/1
  [BRAKE_1_TEMP] -> Cast33/1
  [BRAKE_1_STATUS] -> Cast32/1
  [BRAKE_2_CURRENT] -> Cast31/1
  [BRAKE_2_TEMP] -> Cast30/1
  Cast/1 -> Bus Assignment/2  "FCC1_ACExxxA_WHEEL_POS_1"
  Cast1/1 -> Bus Assignment/3  "FCC1_ACExxxA_WHEEL_POS_1"
  Cast2/1 -> Bus Assignment/4  "FCC1_ACExxxA_WHEEL_POS_1"
  Cast3/1 -> Bus Assignment/5  "FCC1_ACExxxA_WHEEL_POS_1"
  Cast4/1 -> Bus Assignment/6
  Cast5/1 -> Bus Assignment/7  "FCC1_ACExxxA_WHEEL_POS_1"
  Cast6/1 -> Bus Assignment/8  "FCC1_ACExxxA_WHEEL_POS_1"
  Cast7/1 -> Bus Assignment/9  "FCC1_ACExxxA_WHEEL_POS_1"
  Cast8/1 -> Bus Assignment/10  "FCC1_ACExxxA_WHEEL_POS_1"
  Cast9/1 -> Bus Assignment/11  "FCC1_ACExxxA_WHEEL_POS_1"
  Cast10/1 -> Bus Assignment/12  "FCC1_ACExxxA_WHEEL_POS_1"
  Cast11/1 -> Bus Assignment/13  "FCC1_ACExxxA_WHEEL_POS_1"
  Cast12/1 -> Bus Assignment/14  "FCC1_ACExxxA_WHEEL_POS_1"
  Cast13/1 -> Bus Assignment/15  "FCC1_ACExxxA_WHEEL_POS_1"
  Cast14/1 -> Bus Assignment/16  "FCC1_ACExxxA_WHEEL_POS_1"
  Cast15/1 -> Bus Assignment/17  "FCC1_ACExxxA_WHEEL_POS_1"
  Cast22/1 -> Bus Assignment/18  "FCC1_ACExxxA_WHEEL_POS_1"
  Cast23/1 -> Bus Assignment/19  "FCC1_ACExxxA_WHEEL_POS_1"
  Cast24/1 -> Bus Assignment/20  "FCC1_ACExxxA_WHEEL_POS_1"
  Cast25/1 -> Bus Assignment/21  "FCC1_ACExxxA_WHEEL_POS_1"
  Cast26/1 -> Bus Assignment/22  "FCC1_ACExxxA_WHEEL_POS_1"
  Cast27/1 -> Bus Assignment/23  "FCC1_ACExxxA_WHEEL_POS_1"
  Cast16/1 -> Bus Assignment/24  "FCC1_ACExxxA_WHEEL_POS_1"
  Cast17/1 -> Bus Assignment/25  "FCC1_ACExxxA_WHEEL_POS_1"
  Cast18/1 -> Bus Assignment/26  "FCC1_ACExxxA_WHEEL_POS_1"
  Cast19/1 -> Bus Assignment/27  "FCC1_ACExxxA_WHEEL_POS_1"
  Cast20/1 -> Bus Assignment/28  "FCC1_ACExxxA_WHEEL_POS_1"
  Cast21/1 -> Bus Assignment/29  "FCC1_ACExxxA_WHEEL_POS_1"
  Cast28/1 -> Bus Assignment/30  "FCC1_ACExxxA_WHEEL_POS_1"
  Cast29/1 -> Bus Assignment/31  "FCC1_ACExxxA_WHEEL_POS_1"
  Cast34/1 -> Bus Assignment/32  "FCC1_ACExxxA_WHEEL_POS_1"
  Cast30/1 -> Bus Assignment/33  "FCC1_ACExxxA_WHEEL_POS_1"
  Cast31/1 -> Bus Assignment/34  "FCC1_ACExxxA_WHEEL_POS_1"
  Cast32/1 -> Bus Assignment/35  "FCC1_ACExxxA_WHEEL_POS_1"
  Cast33/1 -> Bus Assignment/36  "FCC1_ACExxxA_WHEEL_POS_1"
  Cast35/1 -> Bus Assignment/37  "FCC1_ACExxxA_WHEEL_POS_1"
